simulink model "showflight"  (Simulink 6.6)
settings: Solver=FixedStepDiscrete  StartTime=0.0  StopTime=inf  FixedStep=1/30  RelTol=1e-3
settings Model: Creator=cox  LastModifiedBy=cox  ExtModeAutoUpdateStatusClock=off

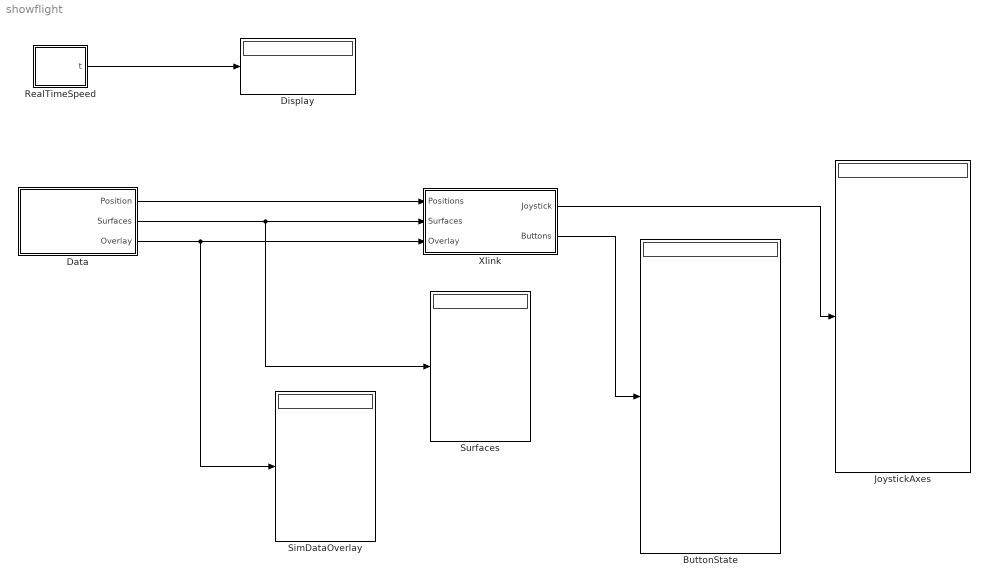
== system showflight ==
  ButtonState : Display
  Data : Subsystem
  Display : Display
  JoystickAxes : Display
  RealTimeSpeed : Subsystem
  SimDataOverlay : Display
  Surfaces : Display
  Xlink : Subsystem  mask(Xlink){HUDCell={'FlightNumber','Time','Elevator','Alpha','Nz','pdeg'}}
      mask prompts: HUDCell "Lables for HUD, (cell array)"
      mask help:
      | Input Positions and Surfaces for X-Plane Visualization.
      |   Positions - [ Latitude, Longitude, Altitude, Roll, Pitch, Yaw] % degrees and ft.
      |   Surfaces  - [ Aileron, Elevator, Rudder, Flaps, Spoiler, GearDown] % deg and 0/1
      |
      | Output is Joysick axes and Button pushes.
      |   Joystick - First 16 axes
      |   Buttons  - 16 buttons as assigned to Xlink in X-Plane
      mask init:
      | if isempty(HUDCell) HUDCell=cell(6,1); end
      | HUDTextArray = uint8(zeros(90,1));
      | 
      | % loop through names, assign to string arrays
      | for i=1:min(length(HUDCell),6);
      |   if length(HUDCell{i})>14 HUDCell{i}=HUDCell{i}(1:14); end
      |   if length(HUDCell{i}>0),
      |     HUDTextArray((i-1)*15+1:(i-1)*15+length(HUDCell{i})) = uint8(HUDCell{i});
      |   end
      | end
  wires:
  RealTimeSpeed/1(t) -> Display/1
  Data/1(Position) -> Xlink/1(Positions)
  Xlink/1(Joystick) -> JoystickAxes/1
  Xlink/2(Buttons) -> ButtonState/1
  Data/2(Surfaces) -> Xlink/2(Surfaces), Surfaces/1
  Data/3(Overlay) -> Xlink/3(Overlay), SimDataOverlay/1

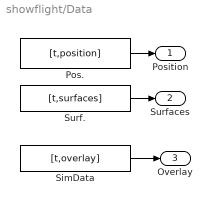
== system showflight/Data ==
  Pos. : FromWorkspace  VariableName=[t,position]  SampleTime=0  OutputAfterFinalValue=Holding final value
  SimData : FromWorkspace  VariableName=[t,overlay]  SampleTime=0  OutputAfterFinalValue=Holding final value
  Surf. : FromWorkspace  VariableName=[t,surfaces]  SampleTime=0  OutputAfterFinalValue=Holding final value
  Position : Outport
  Surfaces : Outport  Port=2
  Overlay : Outport  Port=3
  wires:
  Pos./1 -> Position/1
  Surf./1 -> Surfaces/1
  SimData/1 -> Overlay/1

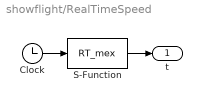
== system showflight/RealTimeSpeed ==
  Clock : Clock
      settings: Decimation=10
  S-Function : S-Function  FunctionName=RT_mex
  t : Outport
  wires:
  S-Function/1 -> t/1
  Clock/1 -> S-Function/1

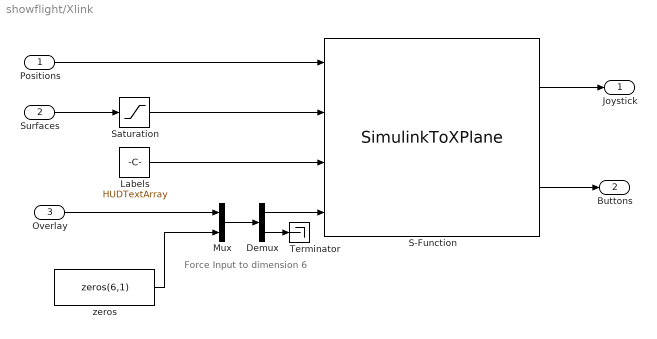
== system showflight/Xlink ==
  note: Force Input to
      | dimension 6
  Positions : Inport
  Surfaces : Inport  Port=2
  Overlay : Inport  Port=3
  Demux : Demux  Outputs=[6 -1]
  Labels : Constant  Value=HUDTextArray  OutDataTypeMode=uint8
  Mux : Mux  Inputs=2
  S-Function : S-Function  FunctionName=SimulinkToXPlane
  Saturation : Saturate  UpperLimit=[180*ones(5,1); 1]  LowerLimit=[-180*ones(5,1); 0]
  Terminator : Terminator
  zeros : Constant  Value=zeros(6,1)  OutDataTypeMode=double
  Joystick : Outport
  Buttons : Outport  Port=2
  wires:
  Positions/1 -> S-Function/1
  S-Function/1 -> Joystick/1
  Surfaces/1 -> Saturation/1
  S-Function/2 -> Buttons/1
  Saturation/1 -> S-Function/2
  Labels/1 -> S-Function/3
  Overlay/1 -> Mux/1
  zeros/1 -> Mux/2
  Mux/1 -> Demux/1
  Demux/1 -> S-Function/4
  Demux/2 -> Terminator/1
